simulink model "frank_differential_drive"  (R2023b)
settings: Solver=VariableStepAuto  StartTime=0.0  StopTime=10  RelTol=1e-3
values from neighbouring files (symbols this model uses):
  qn = [0, pi/4, pi, 0, pi/4, 0]    [OMPro.m]    (also in OMPro_v1.m = [0, -pi/4, 0, 0, pi/4, 0]; OManPro.m = rand(1,6); moron9dof.m = [0.1 0.1 pi/4 pi/4 -pi/4 pi/4 0 pi/4 0])
undefined symbols (not defined in the file or in its folder): cinertia, nofriction, omega_tilde, p560
libraries: roblocks x25, robotmobilelib x3
settings Model: NumberOfSteps=10  Creator=kangwang  LastModifiedBy=kangwang

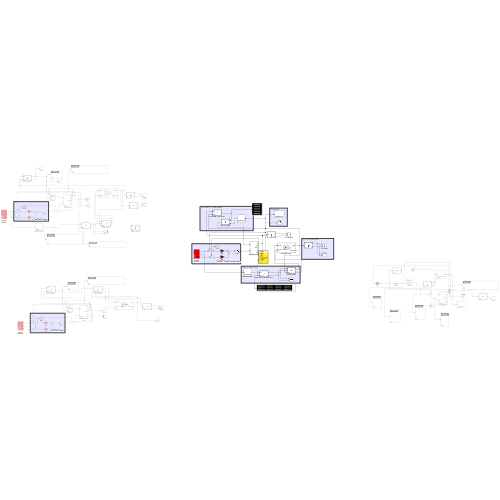
[thumbnail: Simulink's stored preview of the top-level diagram]
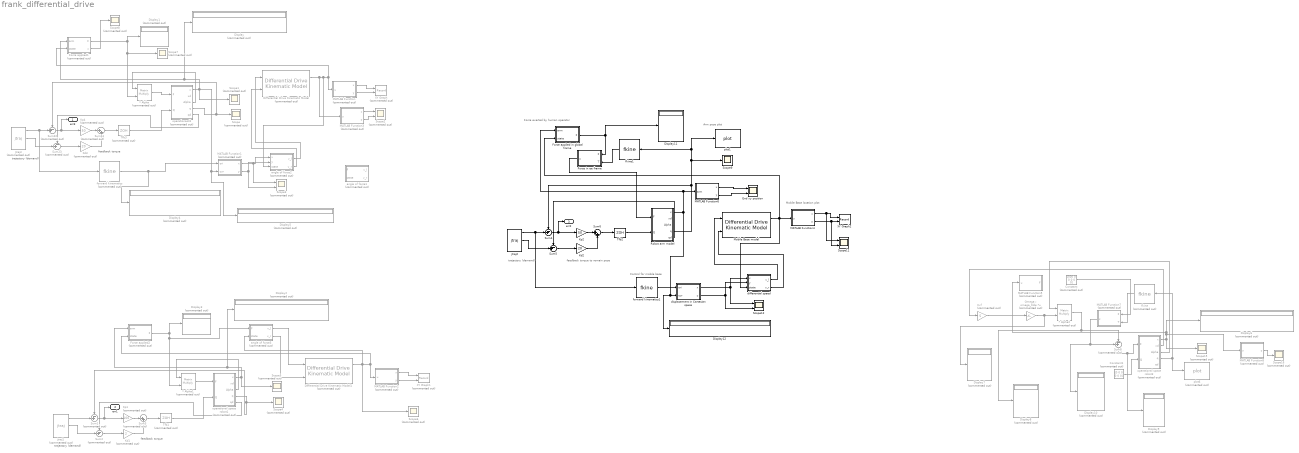
== system frank_differential_drive ==
  note: Mobile Base location plot
  note: Arm pose plot
  note: Control for mobile base
  note: Force exerted by human operator
  note: feedback torque
  note: trajectory
      | (demand)
  note: trajectory
      | (demand)
  note: feedback torque
  note: trajectory
      | (demand)
  note: feedback torque to remain pose
  * Alpha : Product  Commented=on  Multiplication=Matrix(*)
  * Alpha1 : Product  Commented=on  Multiplication=Matrix(*)
  * Alpha2 : Product  Commented=on  Multiplication=Matrix(*)
  Constant : Constant  Commented=on  Value=[500 0 0 0 0 0]
  Constant1 : Constant  Commented=on  Value=[0 0 0 0 0 0]
  Differential Drive Kinematic Model : robotmobilelib/Differential Drive Kinematic Model  Commented=on  VehicleInputs=Wheel Speeds  WheelRadius=0.05  WheelSpeedRange=[-inf inf]  TrackWidth=0.2  InitialState=[0; 0; 0]  SimulateUsing=Interpreted execution
  Differential Drive Kinematic Model1 : robotmobilelib/Differential Drive Kinematic Model  Commented=on  VehicleInputs=Wheel Speeds  WheelRadius=0.05  WheelSpeedRange=[-inf inf]  TrackWidth=0.2  InitialState=[0; 0; 0]  SimulateUsing=Interpreted execution
  Display{,1..10} (11 alike) : Display  Commented=on
  Display11 : Display
  Display12 : Display
  End xy position : Scope  NumInputPorts=2
  Force applied in global frame : MATLAB Function  TreatAsAtomicUnit=on
  Force applied1 : MATLAB Function  Commented=on  TreatAsAtomicUnit=on
  Force applied2 : MATLAB Function  Commented=on  TreatAsAtomicUnit=on
  Force in ee frame : MATLAB Function  TreatAsAtomicUnit=on
  Kd1 : Gain  Commented=on  Gain=2  SaturateOnIntegerOverflow=on  OutDataTypeStr=Inherit: Same as input  ParamDataTypeStr=Inherit: Same as input
  Kd2 : Gain  Gain=20  SaturateOnIntegerOverflow=on  OutDataTypeStr=Inherit: Same as input  ParamDataTypeStr=Inherit: Same as input
  Kd3 : Gain  Commented=on  Gain=20  SaturateOnIntegerOverflow=on  OutDataTypeStr=Inherit: Same as input  ParamDataTypeStr=Inherit: Same as input
  Kp1 : Gain  Commented=on  Gain=100  SaturateOnIntegerOverflow=on  OutDataTypeStr=Inherit: Same as input  ParamDataTypeStr=Inherit: Same as input
  Kp2 : Gain  Gain=50  SaturateOnIntegerOverflow=on  OutDataTypeStr=Inherit: Same as input  ParamDataTypeStr=Inherit: Same as input
  Kp4 : Gain  Commented=on  Gain=50  SaturateOnIntegerOverflow=on  OutDataTypeStr=Inherit: Same as input  ParamDataTypeStr=Inherit: Same as input
  Kvf : Gain  Commented=on  Gain=5
  MATLAB Function : MATLAB Function  Commented=on  TreatAsAtomicUnit=on
  MATLAB Function1 : MATLAB Function  Commented=on  TreatAsAtomicUnit=on
  MATLAB Function2 : MATLAB Function  Commented=on  TreatAsAtomicUnit=on
  MATLAB Function3 : MATLAB Function  Commented=on  TreatAsAtomicUnit=on
  MATLAB Function4 : MATLAB Function  TreatAsAtomicUnit=on
  MATLAB Function5 : MATLAB Function  Commented=on  TreatAsAtomicUnit=on
  MATLAB Function6 : MATLAB Function  TreatAsAtomicUnit=on
  MATLAB Function7 : MATLAB Function  Commented=on  TreatAsAtomicUnit=on
  MATLAB Function8 : MATLAB Function  Commented=on  TreatAsAtomicUnit=on
  Mobile Base model : robotmobilelib/Differential Drive Kinematic Model  VehicleInputs=Wheel Speeds  WheelRadius=0.05  WheelSpeedRange=[-inf inf]  TrackWidth=0.2  InitialState=[0; 0; 0]  SimulateUsing=Interpreted execution
  Omega~ : Gain  Commented=on  Gain=omega_tilde  Multiplication=Matrix(K*u)
  Robot arm model : Subsystem  mask{robot=nofriction(p560), q0=qn}
      mask prompts: q0 "Initial joint angles"
  Scope{,1,4..8,15..16} (9 alike) : Scope  Commented=on
  Scope11 : Scope  NumInputPorts=2
  Scope12 : Scope  NumInputPorts=2
  Scope2 : Scope  Commented=on  NumInputPorts=2
  Scope3 : Scope  Commented=on  NumInputPorts=2
  Scope9 : Scope
  Sum{1..2,22..23} (4 alike) : Sum  Commented=on  Inputs=-+|  InputSameDT=on  SaturateOnIntegerOverflow=on  OutDataTypeStr=Inherit: Same as first input
  Sum24 : Sum  Commented=on  Inputs=|++  InputSameDT=on  SaturateOnIntegerOverflow=on  OutDataTypeStr=Inherit: Same as first input
  Sum3 : Sum  Commented=on  Inputs=|++  InputSameDT=on  SaturateOnIntegerOverflow=on  OutDataTypeStr=Inherit: Same as first input
  Sum4 : Sum  Inputs=-+|  InputSameDT=on  SaturateOnIntegerOverflow=on  OutDataTypeStr=Inherit: Same as first input
  Sum5 : Sum  Inputs=-+|  InputSameDT=on  SaturateOnIntegerOverflow=on  OutDataTypeStr=Inherit: Same as first input
  Sum6 : Sum  Inputs=|++  InputSameDT=on  SaturateOnIntegerOverflow=on  OutDataTypeStr=Inherit: Same as first input
  Sum8 : Sum  Commented=on  Inputs=+-|
  Tfb1 : ZeroOrderHold  Commented=on  SampleTime=0.002
  Tfb2 : ZeroOrderHold  SampleTime=0.002
  Tfb3 : ZeroOrderHold  Commented=on  SampleTime=0.002
  XY Graph : Record  Commented=on  FileSettingsInternal="{\"entries\":[{\"content\":{\"excelSettings\":{\"content\":{},\"type\":\"Streamout.ExcelSettings\"}},\"type\":\"Streamout.FileSettingStorage\",\"uuid\":\"\"}],\"packageUris\":[\"http:\\/\\/schema.mathworks.com\\/mf0\\/streamout_blocks\\/R2020a\"],\"version\":\"1.0\"}"  Layout=[1 1]  SignalsInternal="{\"entries\":[{\"content\":{\"signals\":[{\"content\":{\"blockPath\":[],\"dimensions\":[1],\"domain\":\"\",\"lineColor\":\"#a2142f\",\"plots\":[1],\"port\":1,\"signalID\":301,\"signalName\":\"MATLAB Function:1\"},\"type\":\"RecordBlkView.Signal\",\"uuid\":\"\"},{\"content\":{\"blockPath\":[],\"dimensions\":[1],\"domain\":\"\",\"lineColor\":\"#139fff\",\"plots\":[1],\"port\":2,\"signalID\":304,\"signalName\":\"MATLAB Function:2\"},\"type\":\"RecordBlkView.Signal\",\"uuid\":\"\"}]},\"type\":\"RecordBlkView.InputSignals\",\"uuid\":\"\"}],\"packageUris\":[\"http:\\/\\/schema.mathworks.com\\/mf0\\/streamout_blocks\\/R2020a\"],\"version\":\"1.0\"}"  VisualizationBindings="{\"xyplotplugin\":{\"info\":[{\"series\":[{\"bindingParametersList\":[{\"parameter\":\"X-Axis\",\"signalID\":301,\"signalName\":\"MATLAB Function:1\"},{\"parameter\":\"Y-Axis\",\"signalID\":304,\"signalName\":\"MATLAB Function:2\"}],\"seriesID\":21445}],\"subplotID\":1}]}}"  CompatibilityTag=XY
  XY Graph1 : Record  Commented=on  FileSettingsInternal="{\"entries\":[{\"content\":{\"excelSettings\":{\"content\":{},\"type\":\"Streamout.ExcelSettings\"}},\"type\":\"Streamout.FileSettingStorage\",\"uuid\":\"\"}],\"packageUris\":[\"http:\\/\\/schema.mathworks.com\\/mf0\\/streamout_blocks\\/R2020a\"],\"version\":\"1.0\"}"  Layout=[1 1]  SignalsInternal="{\"entries\":[{\"content\":{\"signals\":[{\"content\":{\"blockPath\":[],\"dimensions\":[1],\"domain\":\"\",\"lineColor\":\"#a2142f\",\"plots\":[1],\"port\":1,\"signalID\":293,\"signalName\":\"MATLAB Function:1\"},\"type\":\"RecordBlkView.Signal\",\"uuid\":\"\"},{\"content\":{\"blockPath\":[],\"dimensions\":[1],\"domain\":\"\",\"lineColor\":\"#139fff\",\"plots\":[1],\"port\":2,\"signalID\":296,\"signalName\":\"MATLAB Function:2\"},\"type\":\"RecordBlkView.Signal\",\"uuid\":\"\"}]},\"type\":\"RecordBlkView.InputSignals\",\"uuid\":\"\"}],\"packageUris\":[\"http:\\/\\/schema.mathworks.com\\/mf0\\/streamout_blocks\\/R2020a\"],\"version\":\"1.0\"}"  VisualizationBindings="{\"xyplotplugin\":{\"info\":[{\"series\":[{\"bindingParametersList\":[{\"parameter\":\"X-Axis\",\"signalID\":293,\"signalName\":\"MATLAB Function:1\"},{\"parameter\":\"Y-Axis\",\"signalID\":296,\"signalName\":\"MATLAB Function:2\"}],\"seriesID\":34754}],\"subplotID\":1}]}}"  CompatibilityTag=XY
  XY Graph2 : Record  FileSettingsInternal="{\"entries\":[{\"content\":{\"excelSettings\":{\"content\":{},\"type\":\"Streamout.ExcelSettings\"}},\"type\":\"Streamout.FileSettingStorage\",\"uuid\":\"\"}],\"packageUris\":[\"http:\\/\\/schema.mathworks.com\\/mf0\\/streamout_blocks\\/R2020a\"],\"version\":\"1.0\"}"  Layout=[1 1]  SignalsInternal="{\"entries\":[{\"content\":{\"signals\":[{\"content\":{\"blockPath\":[],\"dimensions\":[1],\"domain\":\"\",\"lineColor\":\"#64d413\",\"plots\":[1],\"port\":1,\"sid\":[\"\"],\"signalID\":158746,\"signalName\":\"MATLAB Function4:1\"},\"type\":\"RecordBlkView.Signal\",\"uuid\":\"\"},{\"content\":{\"blockPath\":[],\"dimensions\":[1],\"domain\":\"\",\"lineColor\":\"#ff13a6\",\"plots\":[1],\"port\":2,\"sid\":[\"\"],\"signalID\":158750,\"signalName\":\"MATLAB Function4:2\"},\"type\":\"RecordBlkView.Signal\",\"uuid\":\"\"}]},\"type\":\"RecordBlkView.InputSignals\",\"uuid\":\"\"}],\"packageUris\":[\"http:\\/\\/schema.mathworks.com\\/mf0\\/streamout_blocks\\/R2020a\"],\"version\":\"1.0\"}"  VisualizationBindings="{\"xyplotplugin\":{\"info\":[{\"series\":[{\"bindingParametersList\":[{\"parameter\":\"X-Axis\",\"signalID\":158746,\"signalName\":\"MATLAB Function4:1\"},{\"parameter\":\"Y-Axis\",\"signalID\":158750,\"signalName\":\"MATLAB Function4:2\"}],\"seriesID\":52797}],\"subplotID\":1}]}}"  CompatibilityTag=XY
  angle of force1 : MATLAB Function  Commented=on  TreatAsAtomicUnit=on
  angle of force2 : MATLAB Function  Commented=on  TreatAsAtomicUnit=on
  angle of force3 : MATLAB Function  Commented=on  TreatAsAtomicUnit=on
  differential speed : MATLAB Function  TreatAsAtomicUnit=on
  displacement in Cartesian space : MATLAB Function  TreatAsAtomicUnit=on
  fkine : roblocks/Arm/fkine  Commented=on  robot=nofriction(p560)
  fkine1 : roblocks/Arm/fkine  robot=nofriction(p560)
  forward kinematics : roblocks/Arm/fkine  Commented=on  robot=nofriction(p560)
  forward kinematics1 : roblocks/Arm/fkine  robot=nofriction(p560)
  jtraj1 : roblocks/Toolbox/jtraj  Commented=on  q0=[0 0.7854 3.1416 0 0.7854 0]  qf=[0 0.7854 3.1416 0 0.7854 0]  tmax=5  ts=0.02
  jtraj2 : roblocks/Toolbox/jtraj  q0=[0 0.7854 3.1416 0 0.7854 0]  qf=[0 0.7854 3.1416 0 0.7854 0]  tmax=5  ts=0.02
  jtraj3 : roblocks/Toolbox/jtraj  Commented=on  q0=[0 0.7854 3.1416 0 0.7854 0]  qf=[0 0.7854 3.1416 0 0.7854 0]  tmax=5  ts=0.02
  operational space robot1 : Subsystem  Commented=on  mask{robot=nofriction(p560), q0=qn}
      mask prompts: q0 "Initial joint angles"
  operational space robot3 : Subsystem  Commented=on  mask{robot=nofriction(p560), q0=qn}
      mask prompts: q0 "Initial joint angles"
  operationaot3 : Subsystem  Commented=on  mask{robot=nofriction(p560), q0=qn}
      mask prompts: q0 "Initial joint angles"
  plot1 : roblocks/Arm/plot  robot=nofriction(p560)  fps=10  holdplot=on
  plot6 : roblocks/Arm/plot  Commented=on  robot=p560  fps=20  holdplot=on
  err3 : Outport
  err1 : Outport  Port=2
  err2 : Outport  Port=3
  wires:
  Sum23/1 -> Kd3/1
  Tfb3/1 -> operationaot3/2(Q)
  operationaot3/4(q) -> Scope/1, Sum22/1
  Force applied1/1(F) -> Scope7/1, * Alpha/2, Display1/1
  operationaot3/1(x) -> Display5/1, MATLAB Function1/2(cur), Scope1/1, Display/1, Force applied1/1(arm)
  * Alpha/1 -> operationaot3/1(F)
  jtraj3/1 -> forward kinematics/1, Sum22/2
  operationaot3/5(qd) -> Sum23/1
  Kp4/1 -> Sum24/1
  Sum22/1 -> err3/1, Kp4/1
  Sum24/1 -> Tfb3/1
  operationaot3/3(Alpha) -> * Alpha/1
  jtraj3/2 -> Sum23/2
  MATLAB Function/1(x) -> XY Graph/1
  MATLAB Function/2(y) -> XY Graph/2
  Kd3/1 -> Sum24/2
  Differential Drive Kinematic Model/1 -> MATLAB Function3/1(u), Force applied1/2(state), MATLAB Function/1(u), angle of force2/3(state)
  forward kinematics/1 -> Display4/1, MATLAB Function1/1(ori)
  MATLAB Function1/1(x) -> Scope3/1, angle of force2/1(x)
  MATLAB Function1/2(y) -> Scope3/2, angle of force2/2(y)
  angle of force2/1(v_l) -> Differential Drive Kinematic Model/1
  angle of force2/2(v_r) -> Differential Drive Kinematic Model/2
  operational space robot1/5(qd) -> Sum2/1
  Force applied2/1(F) -> angle of force3/1(F), * Alpha1/2, Display3/1
  jtraj1/1 -> Sum1/2
  operational space robot1/3(Alpha) -> * Alpha1/1
  Tfb1/1 -> operational space robot1/2(Q)
  Kp1/1 -> Sum3/1
  operational space robot1/1(x) -> Scope5/1, Display2/1, Force applied2/1(arm)
  * Alpha1/1 -> operational space robot1/1(F)
  Kd1/1 -> Sum3/2
  Differential Drive Kinematic Model1/1 -> Scope6/1, angle of force3/2(state), Force applied2/2(state), MATLAB Function2/1(u)
  Sum3/1 -> Tfb1/1
  operational space robot1/4(q) -> Scope4/1, Sum1/1
  Sum1/1 -> err1/1, Kp1/1
  MATLAB Function2/2(y) -> XY Graph1/2
  Sum2/1 -> Kd1/1
  MATLAB Function2/1(x) -> XY Graph1/1
  jtraj1/2 -> Sum2/2
  angle of force3/1(v_l) -> Differential Drive Kinematic Model1/1
  angle of force3/2(v_r) -> Differential Drive Kinematic Model1/2
  Force applied1/2(x) -> Scope8/1
  MATLAB Function3/1(x) -> Scope2/1
  MATLAB Function3/2(y) -> Scope2/2
  differential speed/1(v_l) -> Mobile Base model/1
  jtraj2/1 -> forward kinematics1/1, Sum4/2
  Robot arm model/5(qd) -> Sum5/1
  Robot arm model/1(x) -> MATLAB Function6/1(arm), Force applied in global frame/1(arm), Display12/1, displacement in Cartesian space/2(cur)
  Tfb2/1 -> Robot arm model/2(Q)
  Kd2/1 -> Sum6/2
  Mobile Base model/1 -> differential speed/3(state), MATLAB Function4/1(u), Force applied in global frame/2(state)
  Sum6/1 -> Tfb2/1
  Sum4/1 -> err2/1, Kp2/1
  MATLAB Function4/2(y) -> Scope11/2, XY Graph2/2
  MATLAB Function4/1(x) -> Scope11/1, XY Graph2/1
  Sum5/1 -> Kd2/1
  jtraj2/2 -> Sum5/2
  displacement in Cartesian space/2(y) -> differential speed/2(y), Scope12/2
  displacement in Cartesian space/1(x) -> differential speed/1(x), Scope12/1
  Kp2/1 -> Sum6/1
  forward kinematics1/1 -> displacement in Cartesian space/1(ori)
  differential speed/2(v_r) -> Mobile Base model/2
  operational space robot3/1(x) -> MATLAB Function5/1(u), Display6/1, MATLAB Function8/1(u), Scope15/1
  operational space robot3/4(q) -> plot6/1, fkine/1
  fkine/1 -> MATLAB Function7/2(T)
  MATLAB Function7/1(c) -> Display10/1, Sum8/1
  MATLAB Function8/1(y) -> Scope16/1
  Force in ee frame/1(c) -> Robot arm model/1(F)
  Robot arm model/4(q) -> plot1/1, fkine1/1, Scope9/1, Sum4/1
  fkine1/1 -> Force in ee frame/2(T)
  Force applied in global frame/1(F) -> Display11/1, Force in ee frame/1(F)
  Constant1/1 -> operational space robot3/2(Q)
  Kvf/1 -> Omega~/1
  * Alpha2/1 -> Display8/1, Sum8/2
  Sum8/1 -> operational space robot3/1(F), Display9/1
  operational space robot3/3(Alpha) -> * Alpha2/1
  Omega~/1 -> Display7/1, * Alpha2/2
  operational space robot3/2(xd) -> Kvf/1
  Constant/1 -> MATLAB Function7/1(F)
  MATLAB Function6/1(x) -> End xy position/1
  MATLAB Function6/2(y) -> End xy position/2

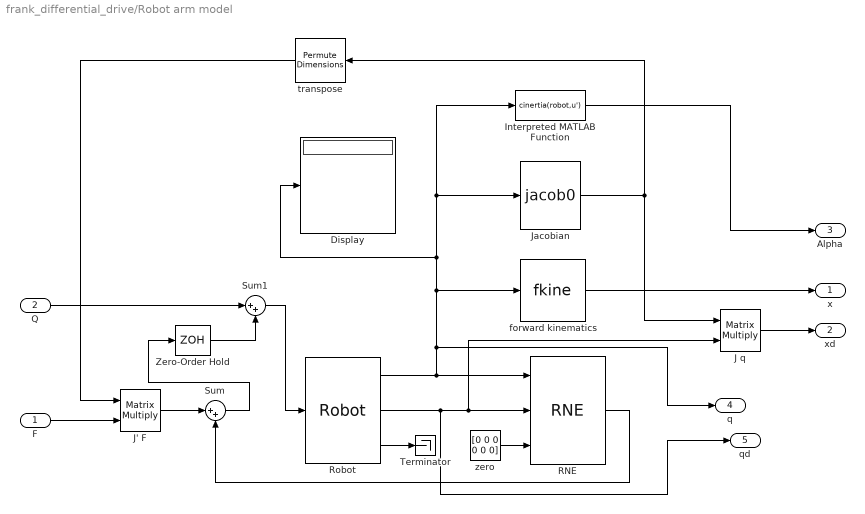
== system frank_differential_drive/Robot arm model ==
  F : Inport
  Q : Inport  Port=2
  Display : Display
  Interpreted MATLAB Function : MATLABFcn  MATLABFcn=cinertia(robot,u')  OutputDimensions=[6 6]  Output1D=off
  J q : Product  Multiplication=Matrix(*)
  J' F : Product  Multiplication=Matrix(*)
  Jacobian : roblocks/Arm/jacob0   robot=robot
  RNE : roblocks/Arm/RNE  robot=robot  grav=[0 0 9.81]
  Robot : roblocks/Arm/Robot  robot=robot  q0=q0
  Sum : Sum  Inputs=|++
  Sum1 : Sum  Inputs=|++
  Terminator : Terminator
  Zero-Order Hold : ZeroOrderHold  SampleTime=5e-3
  forward kinematics : roblocks/Arm/fkine  robot=robot
  transpose : PermuteDimensions
  zero : Constant  Value=[0 0 0 0 0 0]
  x : Outport
  xd : Outport  Port=2
  Alpha : Outport  Port=3
  q : Outport  Port=4
  qd : Outport  Port=5
  wires:
  Interpreted MATLAB Function/1 -> Alpha/1
  Sum/1 -> Zero-Order Hold/1
  F/1 -> J' F/2
  transpose/1 -> J' F/1
  J' F/1 -> Sum/1
  zero/1 -> RNE/3
  Robot/3 -> Terminator/1
  Robot/2 -> qd/1, RNE/2, J q/2
  Robot/1 -> RNE/1, forward kinematics/1, Interpreted MATLAB Function/1, Jacobian/1, Display/1, q/1
  forward kinematics/1 -> x/1
  J q/1 -> xd/1
  Jacobian/1 -> transpose/1, J q/1
  Q/1 -> Sum1/1
  Sum1/1 -> Robot/1
  Zero-Order Hold/1 -> Sum1/2
  RNE/1 -> Sum/2

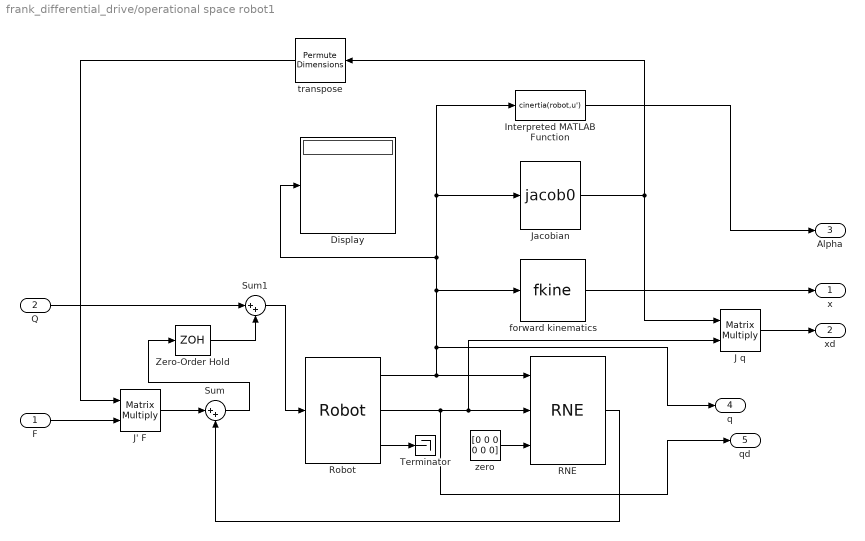
== system frank_differential_drive/operational space robot1 ==
  F : Inport
  Q : Inport  Port=2
  Display : Display
  Interpreted MATLAB Function : MATLABFcn  MATLABFcn=cinertia(robot,u')  OutputDimensions=[6 6]  Output1D=off
  J q : Product  Multiplication=Matrix(*)
  J' F : Product  Multiplication=Matrix(*)
  Jacobian : roblocks/Arm/jacob0   robot=robot
  RNE : roblocks/Arm/RNE  robot=robot  grav=[0 0 9.81]
  Robot : roblocks/Arm/Robot  robot=robot  q0=q0
  Sum : Sum  Inputs=|++
  Sum1 : Sum  Inputs=|++
  Terminator : Terminator
  Zero-Order Hold : ZeroOrderHold  SampleTime=5e-3
  forward kinematics : roblocks/Arm/fkine  robot=robot
  transpose : PermuteDimensions
  zero : Constant  Value=[0 0 0 0 0 0]
  x : Outport
  xd : Outport  Port=2
  Alpha : Outport  Port=3
  q : Outport  Port=4
  qd : Outport  Port=5
  wires:
  Interpreted MATLAB Function/1 -> Alpha/1
  Sum/1 -> Zero-Order Hold/1
  F/1 -> J' F/2
  transpose/1 -> J' F/1
  J' F/1 -> Sum/1
  RNE/1 -> Sum/2
  zero/1 -> RNE/3
  Robot/3 -> Terminator/1
  Robot/2 -> qd/1, RNE/2, J q/2
  Robot/1 -> RNE/1, forward kinematics/1, Interpreted MATLAB Function/1, Jacobian/1, Display/1, q/1
  forward kinematics/1 -> x/1
  J q/1 -> xd/1
  Jacobian/1 -> transpose/1, J q/1
  Q/1 -> Sum1/1
  Sum1/1 -> Robot/1
  Zero-Order Hold/1 -> Sum1/2

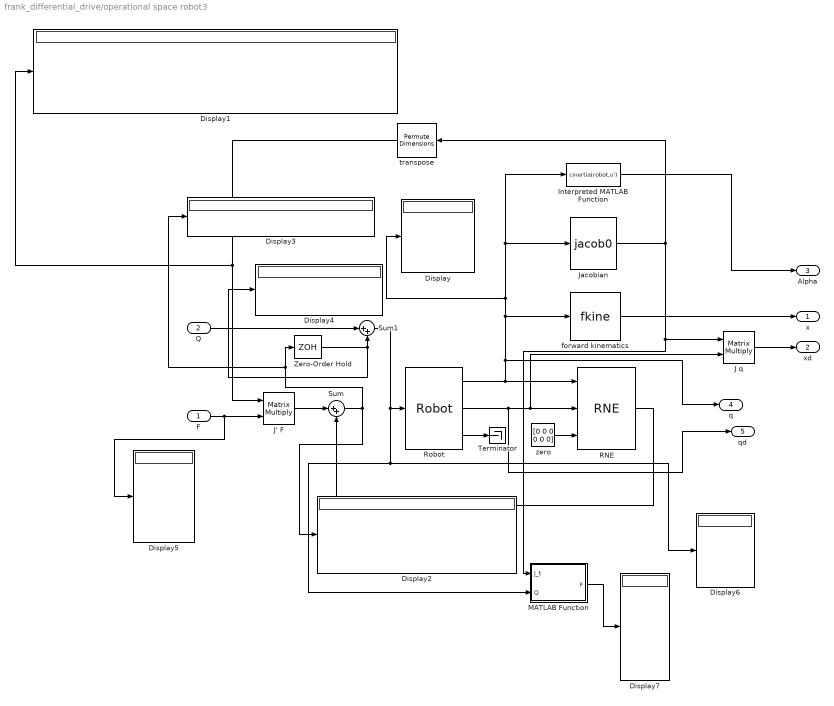
== system frank_differential_drive/operational space robot3 ==
  F : Inport
  Q : Inport  Port=2
  Display{,1..7} (8 alike) : Display
  Interpreted MATLAB Function : MATLABFcn  MATLABFcn=cinertia(robot,u')  OutputDimensions=[6 6]  Output1D=off
  J q : Product  Multiplication=Matrix(*)
  J' F : Product  Multiplication=Matrix(*)
  Jacobian : roblocks/Arm/jacob0   robot=robot
  MATLAB Function : MATLAB Function  TreatAsAtomicUnit=on
  RNE : roblocks/Arm/RNE  robot=robot  grav=[0 0 9.81]
  Robot : roblocks/Arm/Robot  robot=robot  q0=q0
  Sum : Sum  Inputs=|++
  Sum1 : Sum  Inputs=|++
  Terminator : Terminator
  Zero-Order Hold : ZeroOrderHold  SampleTime=5e-3
  forward kinematics : roblocks/Arm/fkine  robot=robot
  transpose : PermuteDimensions
  zero : Constant  Value=[0 0 0 0 0 0]
  x : Outport
  xd : Outport  Port=2
  Alpha : Outport  Port=3
  q : Outport  Port=4
  qd : Outport  Port=5
  wires:
  Interpreted MATLAB Function/1 -> Alpha/1
  Sum/1 -> Display2/1, Zero-Order Hold/1, Display3/1
  F/1 -> Display5/1, J' F/2
  transpose/1 -> Display1/1, J' F/1
  J' F/1 -> Sum/1
  zero/1 -> RNE/3
  Robot/3 -> Terminator/1
  Robot/2 -> qd/1, RNE/2, J q/2
  Robot/1 -> RNE/1, forward kinematics/1, Interpreted MATLAB Function/1, Jacobian/1, Display/1, q/1
  forward kinematics/1 -> x/1
  J q/1 -> xd/1
  Jacobian/1 -> MATLAB Function/1(J_t), J q/1, transpose/1
  Q/1 -> Sum1/1
  Sum1/1 -> MATLAB Function/2(Q), Display6/1, Robot/1
  Zero-Order Hold/1 -> Display4/1, Sum1/2
  RNE/1 -> Sum/2
  MATLAB Function/1(F) -> Display7/1

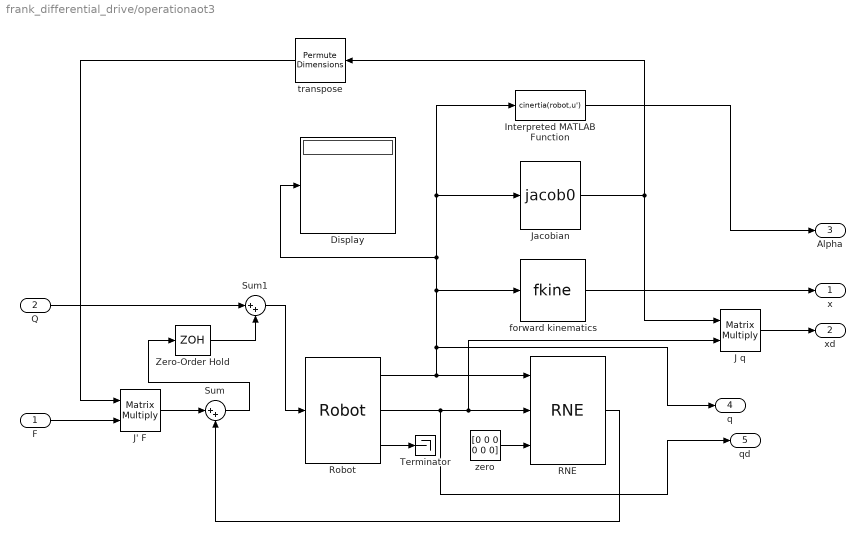
== system frank_differential_drive/operationaot3 ==
  F : Inport
  Q : Inport  Port=2
  Display : Display
  Interpreted MATLAB Function : MATLABFcn  MATLABFcn=cinertia(robot,u')  OutputDimensions=[6 6]  Output1D=off
  J q : Product  Multiplication=Matrix(*)
  J' F : Product  Multiplication=Matrix(*)
  Jacobian : roblocks/Arm/jacob0   robot=robot
  RNE : roblocks/Arm/RNE  robot=robot  grav=[0 0 9.81]
  Robot : roblocks/Arm/Robot  robot=robot  q0=q0
  Sum : Sum  Inputs=|++
  Sum1 : Sum  Inputs=|++
  Terminator : Terminator
  Zero-Order Hold : ZeroOrderHold  SampleTime=5e-3
  forward kinematics : roblocks/Arm/fkine  robot=robot
  transpose : PermuteDimensions
  zero : Constant  Value=[0 0 0 0 0 0]
  x : Outport
  xd : Outport  Port=2
  Alpha : Outport  Port=3
  q : Outport  Port=4
  qd : Outport  Port=5
  wires:
  Interpreted MATLAB Function/1 -> Alpha/1
  Sum/1 -> Zero-Order Hold/1
  F/1 -> J' F/2
  transpose/1 -> J' F/1
  J' F/1 -> Sum/1
  RNE/1 -> Sum/2
  zero/1 -> RNE/3
  Robot/3 -> Terminator/1
  Robot/2 -> qd/1, RNE/2, J q/2
  Robot/1 -> RNE/1, forward kinematics/1, Interpreted MATLAB Function/1, Jacobian/1, Display/1, q/1
  forward kinematics/1 -> x/1
  J q/1 -> xd/1
  Jacobian/1 -> transpose/1, J q/1
  Q/1 -> Sum1/1
  Sum1/1 -> Robot/1
  Zero-Order Hold/1 -> Sum1/2

== matlab function frank_differential_drive/angle of force2 ==
  data: x input; y input; v_l output; v_r output; state input
function [v_l, v_r]= fcn(x, y, state)
current_heading = state(3);           
k_theta = 2.0;                    

r = 0.05;                         
L = 0.2;                          


force_angle = atan2(y, x);
speed = 10*norm([x, y]);

error_theta = wrapToPi(force_angle - current_heading);
w = k_theta * error_theta;

v = speed;  

v_l = (2*v - w*L)/(2*r);
v_r = (2*v + w*L)/(2*r);

== matlab function frank_differential_drive/displacement in Cartesian space ==
  data: x output; ori input; y output; cur input
function [x,y]= fcn(ori, cur)
x = cur(1,4)-ori(1,4);
y = cur(2,4)-ori(2,4);

== matlab function frank_differential_drive/MATLAB Function5 ==
  data: u input; F output
function F = fcn(u)
x = u(1,4);
y = u(2,4);
F = [5 5 0 0 0 0 ].';
if x>1.5 && y > 1.5
    F = [0 0 0 0 0 0].';
end

== matlab function frank_differential_drive/Force applied in global frame ==
  data: arm input; F output; state input
function F = fcn(arm,state)
x_arm = arm(1,4);
x_base = state(1);
y_arm = arm(2,4);
y_base = state(2);
x = x_base+x_arm
y = y_base+y_arm
F = [0 0 0 0 0 0].';
if x<1.8 || y<1.8 
    F = [5 5 0 0 0 0].';
end

== matlab function frank_differential_drive/differential speed ==
  data: x input; y input; v_l output; v_r output; state input
function [v_l, v_r]= fcn(x, y, state)
    current_heading = state(3);           
    k_theta = 2.0;                    

    r = 0.05;                         
    L = 0.2;                          

    % Rebalancing y-direction influence
    y_scale = 0.522;  % Try values < 1 to reduce y influence
    y_scale = 1.0;  % Try values < 1 to reduce y influence
    x_scale = 1.0;  % Keep x unchanged (or tweak as needed)

    x_scaled = x_scale * x;
    y_scaled = y_scale * y;

    force_angle = atan2(y_scaled, x_scaled);

    % gain for the speed (also using scaled values)
    speed = 10 * norm([x_scaled, y_scaled]);

    error_theta = wrapToPi(force_angle - current_heading);
    w = k_theta * error_theta;

    v = speed;  

    v_l = (2*v - w*L)/(2*r);
    v_r = (2*v + w*L)/(2*r);
end

== matlab function frank_differential_drive/MATLAB Function7 ==
  data: F input; T input; c output
function c = fcn(F, T)
y = inv(T(1:3,1:3))*F(1:3)
c = [y.', 0,0,0].'

== matlab function frank_differential_drive/MATLAB Function8 ==
  data: u input; y output
function y = fcn(u)

y = u(1:3,4);

== matlab function frank_differential_drive/operational space robot3/MATLAB Function ==
  data: J_t input; F output; Q input
function F = fcn(J_t,Q)

F = inv(J_t)*Q;

== matlab function frank_differential_drive/MATLAB Function6 ==
  data: x output; arm input; y output
function [x,y]= fcn(arm)
x = arm(1,4);
y = arm(2,4);

== matlab function frank_differential_drive/MATLAB Function1 ==
  data: x output; ori input; y output; cur input
function [x,y]= fcn(ori, cur)
x = cur(1,4)-ori(1,4);
y = cur(2,4)-ori(2,4);

== matlab function frank_differential_drive/Force applied2 ==
  data: arm input; F output; state input
function F = fcn(arm,state)
x_arm = arm(1,4);
x_base = state(1);
x = x_base+x_arm;
F = [0 0 0 0 0 0].';
if x < 1.8 
    F = [5 0 0 0 0 0].';
end

== matlab function frank_differential_drive/MATLAB Function2 ==
  data: x output; u input; y output
function [x,y]= fcn(u)

x = u(1);
y = u(2);

== matlab function frank_differential_drive/MATLAB Function3 ==
  data: x output; u input; y output
function [x,y]= fcn(u)
x = u(1)
y = u(2);

== matlab function frank_differential_drive/Force applied1 ==
  data: arm input; F output; state input; x output
function [F,x]= fcn(arm,state)
x_arm = arm(1,4);
x_base = state(1);
x = x_base+x_arm;
F = [0 0 0 0 0 0].';
if x < 1.8 
    F = [5 0 0 0 0 0].';
end

== matlab function frank_differential_drive/angle of force1 ==
  data: F input; v_l output; v_r output; state input
function [v_l, v_r]= fcn(F, state)
current_heading = state(3);           
k_theta = 2.0;                    

r = 0.05;                         
L = 0.2;                          

Fx = F(1);
Fy = F(2);
force_angle = atan2(Fy, Fx);
speed = norm([Fx, Fy]);

error_theta = wrapToPi(force_angle - current_heading);
w = k_theta * error_theta;

v = speed;  

v_l = (2*v - w*L)/(2*r);
v_r = (2*v + w*L)/(2*r);

== matlab function frank_differential_drive/MATLAB Function ==
  data: x output; u input; y output
function [x,y]= fcn(u)

x = u(1);
y = u(2);

== matlab function frank_differential_drive/angle of force3 ==
  data: F input; v_l output; v_r output; state input
function [v_l, v_r]= fcn(F, state)
current_heading = state(3);           
k_theta = 2.0;                    

r = 0.05;                         
L = 0.2;                          

Fx = F(1);
Fy = F(2);
force_angle = atan2(Fy, Fx);
speed = norm([Fx, Fy]);

error_theta = wrapToPi(force_angle - current_heading);
w = k_theta * error_theta;

v = speed;  

v_l = (2*v - w*L)/(2*r);
v_r = (2*v + w*L)/(2*r);

== matlab function frank_differential_drive/Force in ee frame ==
  data: F input; T input; c output
function c = fcn(F, T)
y = inv(T(1:3,1:3))*F(1:3);
c = [y.', 0,0,0].';

== matlab function frank_differential_drive/MATLAB Function4 ==
  data: x output; u input; y output
function [x,y]= fcn(u)

x = u(1);
y = u(2);
